simulink model "Full_drone_1_2"  (R2020b)
settings: Solver=VariableStepAuto  StartTime=0.0  StopTime=10  RelTol=1e-3
model workspace: external: MATLAB File C:\Users\maria\MATLAB\Projects\untitled\simscape_test\Full_drone_1_2_DataFile.m (data not in the file)
undefined symbols (not defined in the file or in its folder): b, CTgain, density, diameter, Jm, Ke, Kt, L, pitchKd, pitchKi, pitchKp, Rm, rollKd, rollKi, rollKp, smiData, X, xKd, xKi, xKp, xRef, Y, yawKd, yawKi, yawKp, yawRef, yKd, yKi, yKp, yRef, Z, zKd, zKi, zKp, zRef
libraries: sm_lib x75, fl_lib x23, nesl_utility x11
(part 1 of 2)
settings Model: Creator=jbmic  LastModifiedBy=maria

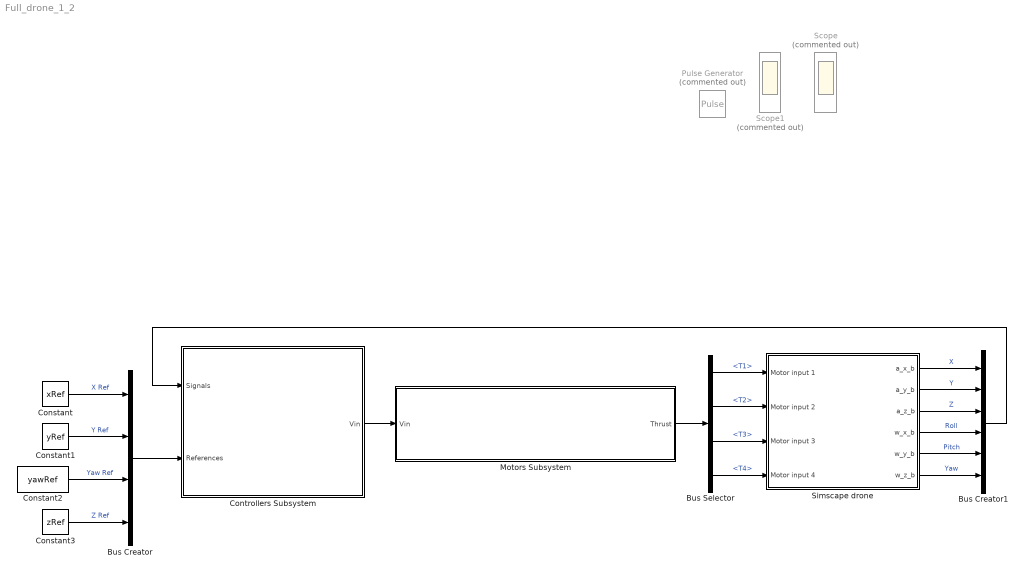
== system Full_drone_1_2 ==
  Bus Creator : BusCreator  Inputs=4
  Bus Creator1 : BusCreator  Inputs=6
  Bus Selector : BusSelector  OutputSignals=T1,T2,T3,T4
  Constant : Constant  Value=xRef
  Constant1 : Constant  Value=yRef
  Constant2 : Constant  Value=yawRef
  Constant3 : Constant  Value=zRef
  Controllers Subsystem : Subsystem
  Motors Subsystem : Subsystem
  Pulse Generator : DiscretePulseGenerator  Commented=on  PulseType=Time based  Amplitude=2  Period=1  PulseWidth=70
  Scope : Scope  Commented=on  NumInputPorts=3
  Scope1 : Scope  Commented=on  NumInputPorts=3
  Simscape drone : Subsystem
  wires:
  Simscape drone/4(w_x_b) -> Bus Creator1/4  "Roll"
  Simscape drone/5(w_y_b) -> Bus Creator1/5  "Pitch"
  Simscape drone/6(w_z_b) -> Bus Creator1/6  "Yaw"
  Simscape drone/3(a_z_b) -> Bus Creator1/3  "Z"
  Simscape drone/2(a_y_b) -> Bus Creator1/2  "Y"
  Simscape drone/1(a_x_b) -> Bus Creator1/1  "X"
  Bus Creator1/1 -> Controllers Subsystem/1(Signals)
  Constant/1 -> Bus Creator/1  "X Ref"
  Constant1/1 -> Bus Creator/2  "Y Ref"
  Constant2/1 -> Bus Creator/3  "Yaw Ref"
  Constant3/1 -> Bus Creator/4  "Z Ref"
  Bus Creator/1 -> Controllers Subsystem/2(References)
  Controllers Subsystem/1(Vin) -> Motors Subsystem/1(Vin)
  Motors Subsystem/1(Thrust) -> Bus Selector/1
  Bus Selector/3 -> Simscape drone/3(Motor input 3)  "<T3>"
  Bus Selector/4 -> Simscape drone/4(Motor input 4)  "<T4>"
  Bus Selector/2 -> Simscape drone/2(Motor input 2)  "<T2>"
  Bus Selector/1 -> Simscape drone/1(Motor input 1)  "<T1>"

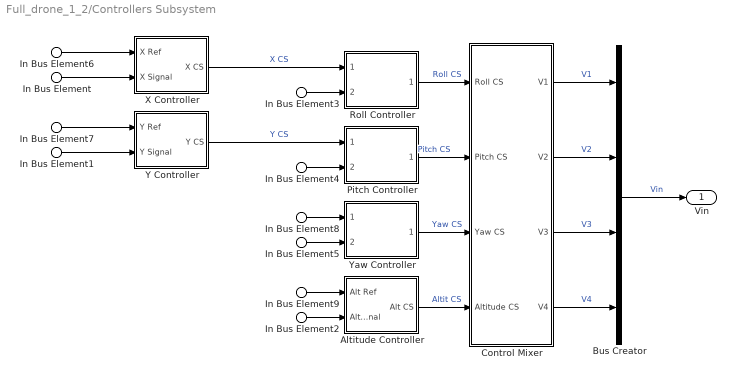
== system Full_drone_1_2/Controllers Subsystem ==
  In Bus Element : Inport  PortName=Signals  Element=X
  In Bus Element1 : Inport  PortName=Signals  Element=Y
  In Bus Element2 : Inport  PortName=Signals  Element=Z
  In Bus Element3 : Inport  PortName=Signals  Element=Roll
  In Bus Element4 : Inport  PortName=Signals  Element=Pitch
  In Bus Element5 : Inport  PortName=Signals  Element=Yaw
  In Bus Element6 : Inport  Port=2  PortName=References  Element=X Ref
  In Bus Element7 : Inport  Port=2  PortName=References  Element=Y Ref
  In Bus Element8 : Inport  Port=2  PortName=References  Element=Yaw Ref
  In Bus Element9 : Inport  Port=2  PortName=References  Element=Z Ref
  Altitude Controller : Subsystem
  Bus Creator : BusCreator  Inputs=4
  Control Mixer : Subsystem
  Pitch Controller : Subsystem
  Roll Controller : Subsystem
  X Controller : Subsystem
  Y Controller : Subsystem
  Yaw Controller : Subsystem
  Vin : Outport
  wires:
  In Bus Element9/1 -> Altitude Controller/1(Alt Ref)
  In Bus Element6/1 -> X Controller/1(X Ref)
  Control Mixer/3(V3) -> Bus Creator/3  "V3"
  In Bus Element8/1 -> Yaw Controller/1(Yaw Ref)
  Yaw Controller/1(Yaw CS) -> Control Mixer/3(Yaw CS)  "Yaw CS"
  In Bus Element7/1 -> Y Controller/1(Y Ref)
  Altitude Controller/1(Alt CS) -> Control Mixer/4(Altitude CS)  "Altit CS"
  X Controller/1(X CS) -> Roll Controller/1(Roll Ref)  "X CS"
  Y Controller/1(Y CS) -> Pitch Controller/1(Pitch Ref)  "Y CS"
  Pitch Controller/1(Pitch CS) -> Control Mixer/2(Pitch CS)  "Pitch CS"
  Control Mixer/2(V2) -> Bus Creator/2  "V2"
  Roll Controller/1(Roll CS) -> Control Mixer/1(Roll CS)  "Roll CS"
  Bus Creator/1 -> Vin/1  "Vin"
  Control Mixer/4(V4) -> Bus Creator/4  "V4"
  Control Mixer/1(V1) -> Bus Creator/1  "V1"
  In Bus Element/1 -> X Controller/2(X Signal)
  In Bus Element1/1 -> Y Controller/2(Y Signal)
  In Bus Element2/1 -> Altitude Controller/2(Alt Signal)
  In Bus Element3/1 -> Roll Controller/2(Roll Signal)
  In Bus Element4/1 -> Pitch Controller/2(Pitch Signal)
  In Bus Element5/1 -> Yaw Controller/2(Yaw Signal)

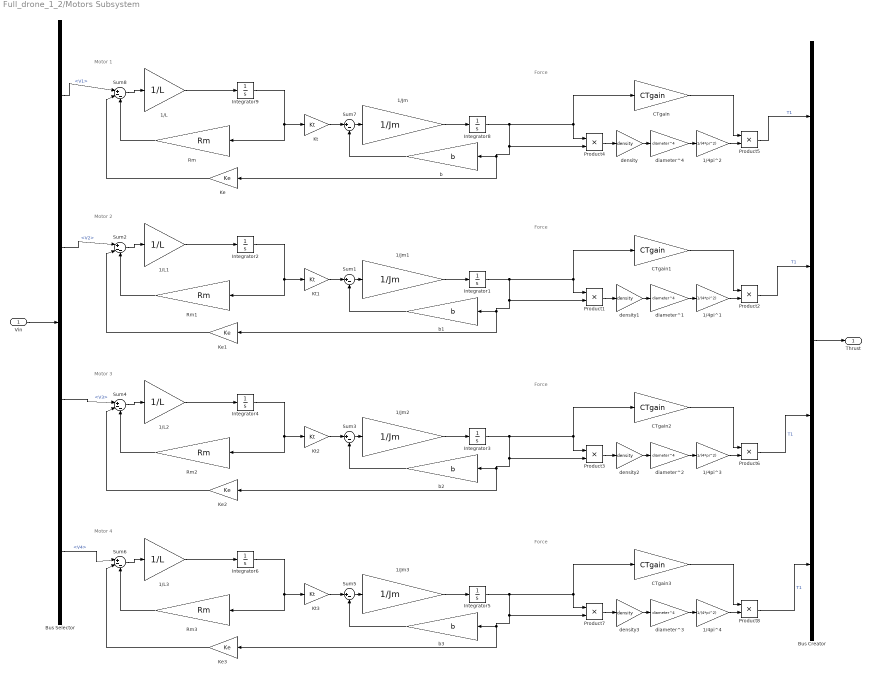
== system Full_drone_1_2/Motors Subsystem ==
  note: Motor 1
  note: Force
  note: Motor 2
  note: Force
  note: Motor 3
  note: Force
  note: Motor 4
  note: Force
  Vin : Inport
  1/4pi^{1..4} (4 alike) : Gain  Gain=1/(4*pi^2)
  1/Jm{,1..3} (4 alike) : Gain  Gain=1/Jm
  1/L{,1..3} (4 alike) : Gain  Gain=1/L
  Bus Creator : BusCreator  Inputs=4
  Bus Selector : BusSelector  OutputSignals=V1,V2,V3,V4
  CTgain{,1..3} (4 alike) : Gain  Gain=CTgain
  Integrator{1..6,8..9} (8 alike) : Integrator
  Ke{,1..3} (4 alike) : Gain  Gain=Ke
  Kt{,1..3} (4 alike) : Gain  Gain=Kt
  Product{1..8} (8 alike) : Product
  Rm{,1..3} (4 alike) : Gain  Gain=Rm
  Sum{1,3,5,7} (4 alike) : Sum  Inputs=|+-
  Sum{2,4,6,8} (4 alike) : Sum  Inputs=|+--
  b{,1..3} (4 alike) : Gain  Gain=b
  density{,1..3} (4 alike) : Gain  Gain=density
  diameter^{1..4} (4 alike) : Gain  Gain=diameter^4
  Thrust : Outport
  wires:
  Rm/1 -> Sum8/3
  1/L/1 -> Integrator9/1
  Sum7/1 -> 1/Jm/1
  density/1 -> diameter^4/1
  Integrator8/1 -> Ke/1, b/1, Product4/2, Product4/1, CTgain/1
  diameter^4/1 -> 1/4pi^2/1
  Ke/1 -> Sum8/2
  Product4/1 -> density/1
  Integrator9/1 -> Kt/1, Rm/1
  1/4pi^2/1 -> Product5/2
  Product5/1 -> Bus Creator/1  "T1"
  Bus Selector/1 -> Sum8/1  "<V1>"
  Sum8/1 -> 1/L/1
  Kt/1 -> Sum7/1
  1/Jm/1 -> Integrator8/1
  CTgain/1 -> Product5/1
  b/1 -> Sum7/2
  Vin/1 -> Bus Selector/1
  Bus Creator/1 -> Thrust/1
  Kt1/1 -> Sum1/1
  1/4pi^1/1 -> Product2/2
  diameter^1/1 -> 1/4pi^1/1
  1/L1/1 -> Integrator2/1
  Integrator1/1 -> Ke1/1, b1/1, Product1/2, Product1/1, CTgain1/1
  Product1/1 -> density1/1
  Ke1/1 -> Sum2/2
  Integrator2/1 -> Kt1/1, Rm1/1
  Sum2/1 -> 1/L1/1
  b1/1 -> Sum1/2
  CTgain1/1 -> Product2/1
  1/Jm1/1 -> Integrator1/1
  density1/1 -> diameter^1/1
  Rm1/1 -> Sum2/3
  Sum1/1 -> 1/Jm1/1
  Bus Selector/2 -> Sum2/1  "<V2>"
  Product2/1 -> Bus Creator/2  "T1"
  Kt2/1 -> Sum3/1
  1/4pi^3/1 -> Product6/2
  diameter^2/1 -> 1/4pi^3/1
  1/L2/1 -> Integrator4/1
  Integrator3/1 -> Ke2/1, b2/1, Product3/2, Product3/1, CTgain2/1
  Product3/1 -> density2/1
  Ke2/1 -> Sum4/2
  Integrator4/1 -> Kt2/1, Rm2/1
  Sum4/1 -> 1/L2/1
  b2/1 -> Sum3/2
  CTgain2/1 -> Product6/1
  1/Jm2/1 -> Integrator3/1
  density2/1 -> diameter^2/1
  Rm2/1 -> Sum4/3
  Sum3/1 -> 1/Jm2/1
  Bus Selector/3 -> Sum4/1  "<V3>"
  Product6/1 -> Bus Creator/3  "T1"
  Kt3/1 -> Sum5/1
  1/4pi^4/1 -> Product8/2
  diameter^3/1 -> 1/4pi^4/1
  1/L3/1 -> Integrator6/1
  Integrator5/1 -> Ke3/1, b3/1, Product7/2, Product7/1, CTgain3/1
  Product7/1 -> density3/1
  Ke3/1 -> Sum6/2
  Integrator6/1 -> Kt3/1, Rm3/1
  Sum6/1 -> 1/L3/1
  b3/1 -> Sum5/2
  CTgain3/1 -> Product8/1
  1/Jm3/1 -> Integrator5/1
  density3/1 -> diameter^3/1
  Rm3/1 -> Sum6/3
  Sum5/1 -> 1/Jm3/1
  Bus Selector/4 -> Sum6/1  "<V4>"
  Product8/1 -> Bus Creator/4  "T1"

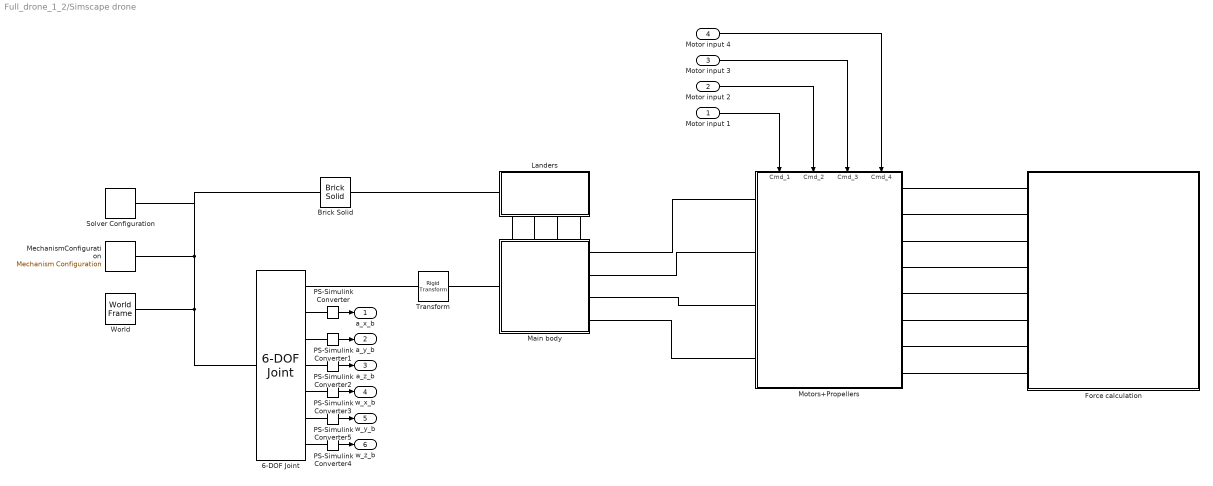
== system Full_drone_1_2/Simscape drone ==
  Motor input 1 : Inport
  Motor input 2 : Inport  Port=2
  Motor input 3 : Inport  Port=3
  Motor input 4 : Inport  Port=4
  6-DOF Joint : sm_lib/Joints/6-DOF Joint  JointMode=Normal  SenseConstraintForce=off  SenseConstraintForceX=off  SenseConstraintForceY=off  SenseConstraintForceZ=off  SenseConstraintTorque=off  SenseConstraintTorqueX=off  SenseConstraintTorqueY=off  SenseConstraintTorqueZ=off  SenseTotalForce=off  SenseTotalForceX=off  SenseTotalForceY=off  SenseTotalForceZ=off  SenseTotalTorque=off  SenseTotalTorqueX=off  SenseTotalTorqueY=off  SenseTotalTorqueZ=off  CompositeWrenchDir=FollowerOnBase  CompositeWrenchFrame=BaseFrame  PxEquilibriumPosition=0  PxEquilibriumPositionUnits=m  PxSpringStiffness=0  PxSpringStiffnessUnits=N/m  PxDampingCoefficient=0  PxDampingCoefficientUnits=N/(m/s)  PxTorqueActuationMode=NoTorque  PxMotionActuationMode=ComputedMotion  PxSensePosition=off  PxSenseVelocity=off  PxSenseAcceleration=on  PxSenseTorqueForce=off  PxSenseLowerLimitTorqueForce=off  PxSenseUpperLimitTorqueForce=off  PxLowerLimitSpecify=off  PxLowerLimitBound=-1  PxLowerLimitBoundUnits=m  PxLowerLimitStiffness=1e6  PxLowerLimitStiffnessUnits=N/m  PxLowerLimitDamping=1e3  PxLowerLimitDampingUnits=N/(m/s)  PxLowerLimitTransitionRegionWidth=1e-4  PxLowerLimitTransitionRegionWidthUnits=m  PxUpperLimitSpecify=off  PxUpperLimitBound=1  PxUpperLimitBoundUnits=m  PxUpperLimitStiffness=1e6  PxUpperLimitStiffnessUnits=N/m  PxUpperLimitDamping=1e3  PxUpperLimitDampingUnits=N/(m/s)  PxUpperLimitTransitionRegionWidth=1e-4  PxUpperLimitTransitionRegionWidthUnits=m  PxPositionTargetSpecify=off  PxPositionTargetPriority=High  PxPositionTargetValue=0  PxPositionTargetValueUnits=m  PxVelocityTargetSpecify=off  PxVelocityTargetPriority=High  PxVelocityTargetValue=0  PxVelocityTargetValueUnits=m/s  PyEquilibriumPosition=0  PyEquilibriumPositionUnits=m  PySpringStiffness=0  PySpringStiffnessUnits=N/m  PyDampingCoefficient=0  PyDampingCoefficientUnits=N/(m/s)  PyTorqueActuationMode=NoTorque  PyMotionActuationMode=ComputedMotion  PySensePosition=off  PySenseVelocity=off  PySenseAcceleration=on  PySenseTorqueForce=off  PySenseLowerLimitTorqueForce=off  PySenseUpperLimitTorqueForce=off  PyLowerLimitSpecify=off  PyLowerLimitBound=0  PyLowerLimitBoundUnits=m  PyLowerLimitStiffness=1e6  PyLowerLimitStiffnessUnits=N/m  PyLowerLimitDamping=1  PyLowerLimitDampingUnits=N/(m/s)  PyLowerLimitTransitionRegionWidth=1e4  PyLowerLimitTransitionRegionWidthUnits=m  PyUpperLimitSpecify=off  PyUpperLimitBound=1  PyUpperLimitBoundUnits=m  PyUpperLimitStiffness=1e6  PyUpperLimitStiffnessUnits=N/m  PyUpperLimitDamping=1e3  PyUpperLimitDampingUnits=N/(m/s)  PyUpperLimitTransitionRegionWidth=1e-4  PyUpperLimitTransitionRegionWidthUnits=m  PyPositionTargetSpecify=off  PyPositionTargetPriority=High  PyPositionTargetValue=0  PyPositionTargetValueUnits=m  PyVelocityTargetSpecify=off  PyVelocityTargetPriority=High  PyVelocityTargetValue=0  PyVelocityTargetValueUnits=m/s  PzEquilibriumPosition=0  PzEquilibriumPositionUnits=m  PzSpringStiffness=0  PzSpringStiffnessUnits=N/m  PzDampingCoefficient=0  PzDampingCoefficientUnits=N/(m/s)  PzTorqueActuationMode=NoTorque  PzMotionActuationMode=ComputedMotion  PzSensePosition=off  PzSenseVelocity=off  PzSenseAcceleration=on  PzSenseTorqueForce=off  PzSenseLowerLimitTorqueForce=off  PzSenseUpperLimitTorqueForce=off  PzLowerLimitSpecify=off  PzLowerLimitBound=-1  PzLowerLimitBoundUnits=m  PzLowerLimitStiffness=1e6  PzLowerLimitStiffnessUnits=N/m  PzLowerLimitDamping=1e3  PzLowerLimitDampingUnits=N/(m/s)  PzLowerLimitTransitionRegionWidth=1e-4  PzLowerLimitTransitionRegionWidthUnits=m  PzUpperLimitSpecify=off  PzUpperLimitBound=1  PzUpperLimitBoundUnits=m  PzUpperLimitStiffness=1e6  PzUpperLimitStiffnessUnits=N/m  PzUpperLimitDamping=1e3  PzUpperLimitDampingUnits=N/(m/s)  PzUpperLimitTransitionRegionWidth=1e-4  PzUpperLimitTransitionRegionWidthUnits=m  PzPositionTargetSpecify=off  PzPositionTargetPriority=High  PzPositionTargetValue=0  PzPositionTargetValueUnits=m  PzVelocityTargetSpecify=off  PzVelocityTargetPriority=High  PzVelocityTargetValue=0  PzVelocityTargetValueUnits=m/s  SphDefPosRotationMethod=None  SphDefPosRotationAngleUnits=deg  SphDefPosRotationStandardAxis=+Z  SphDefPosRotationAngle=0.0  SphDefPosRotationArbitraryAxis=[0 0 1]  SphDefPosFollAlignAxisA=+X  SphDefPosBaseAlignAxisA=+Y  SphDefPosFollAlignAxisB=+Y  SphDefPosBaseAlignAxisB=+Z  SphDefPosRotationSequenceAxes=FollowerAxes  SphDefPosRotationSequence=XYX  SphDefPosRotationSequenceAngles=[0 0 0]  SphDefPosRotationSequenceAnglesUnits=deg  SphDefPosRotationMatrix=[1 0 0; 0 1 0; 0 0 1]  SphEqPosRotationMethod=None  SphEqPosRotationAngleUnits=deg  SphEqPosRotationStandardAxis=+Z  SphEqPosRotationAngle=0.0  SphEqPosRotationArbitraryAxis=[0 0 1]  SphEqPosFollAlignAxisA=+X  SphEqPosBaseAlignAxisA=+Y  SphEqPosFollAlignAxisB=+Y  SphEqPosBaseAlignAxisB=+Z  SphEqPosRotationSequenceAxes=FollowerAxes  SphEqPosRotationSequence=XYX  SphEqPosRotationSequenceAngles=[0 0 0]  SphEqPosRotationSequenceAnglesUnits=deg  SphEqPosRotationMatrix=[1 0 0; 0 1 0; 0 0 1]  SphSpringStiffness=0  SphSpringStiffnessUnits=N*m/deg  SphDampingCoefficient=1e-2  SphDampingCoefficientUnits=N*m/(deg/s)  SphActuateTorqueX=off  SphActuateTorqueY=off  SphActuateTorqueZ=off  SphActuateTorque=off  SphTorqueActuationMode=NoTorque  SphMotionActuationMode=ComputedMotion  SphActuationFrame=BaseFrame  SphSensePosition=off  SphSenseVelocityX=on  SphSenseVelocityY=on  SphSenseVelocityZ=on  SphSenseVelocity=off  SphSenseAccelerationX=off  SphSenseAccelerationY=off  SphSenseAccelerationZ=off  SphSenseAcceleration=off  SphSenseTorqueX=off  SphSenseTorqueY=off  SphSenseTorqueZ=off  SphSenseTorqueForce=off  SphSenseLowerLimitTorqueMag=off  SphSenseUpperLimitTorqueMag=off  SphSensingFrame=BaseFrame  SphLowerLimitSpecify=off  SphLowerLimitBound=15  SphLowerLimitBoundUnits=deg  SphLowerLimitStiffness=1e4  SphLowerLimitStiffnessUnits=N*m/deg  SphLowerLimitDamping=10  SphLowerLimitDampingUnits=N*m/(deg/s)  SphLowerLimitTransitionRegionWidth=0.1  SphLowerLimitTransitionRegionWidthUnits=deg  SphUpperLimitSpecify=off  SphUpperLimitBound=45  SphUpperLimitBoundUnits=deg  SphUpperLimitStiffness=1e4  SphUpperLimitStiffnessUnits=N*m/deg  SphUpperLimitDamping=10  SphUpperLimitDampingUnits=N*m/(deg/s)  SphUpperLimitTransitionRegionWidth=0.1  SphUpperLimitTransitionRegionWidthUnits=deg  SphPositionTargetRotationMethod=None  SphPositionTargetRotationAngleUnits=deg  SphPositionTargetRotationStandardAxis=+Z  SphPositionTargetRotationAngle=0.0  SphPositionTargetRotationArbitraryAxis=[0 0 1]  SphPositionTargetFollAlignAxisA=+X  SphPositionTargetBaseAlignAxisA=+Y  SphPositionTargetFollAlignAxisB=+Y  SphPositionTargetBaseAlignAxisB=+Z  SphPositionTargetRotationSequenceAxes=FollowerAxes  SphPositionTargetRotationSequence=XYX  SphPositionTargetRotationSequenceAngles=[0 0 0]  SphPositionTargetRotationSequenceAnglesUnits=deg  SphPositionTargetRotationMatrix=[1 0 0; 0 1 0; 0 0 1]  SphPositionTargetSpecify=off  SphPositionTargetPriority=High  SphVelocityTargetValue=[0 0 0]  SphVelocityTargetValueUnits=deg/s  SphVelocityTargetSpecify=off  SphVelocityTargetPriority=High  SphVelocityTargetInFollowerFrame=on
  Brick Solid : sm_lib/Body Elements/Brick Solid  GraphicAmbientColor=[0.15 0.15 0.15 1.0]  BasedOnType=Density  BrickDimensions=[1 1 0.002]  BrickDimensionUnits=m  CenterOfMass=[0 0 0]  CenterOfMassUnits=m  GraphicDiffuseColor=[0.5 0.5 0.5]  Density=1000  DensityUnits=kg/m^3  DoExposeReferenceFrame=on  GraphicEmissiveColor=[0.0 0.0 0.0 1.0]  ExportEntireGeometry=on  SerializedFrames=<Frames/>  MarkerShape=Sphere  MarkerSize=10  GraphicType=FromGeometry  InertiaType=CalculateFromGeometry  Mass=1  MassUnits=kg  MomentsOfInertia=[1 1 1]  MomentsOfInertiaUnits=kg*m^2  GraphicOpacity=1.0  ProductsOfInertia=[0 0 0]  ProductsOfInertiaUnits=kg*m^2  GraphicShininess=75  GraphicSpecularColor=[0.5 0.5 0.5 1.0]  GraphicVisPropType=SimpleVisualProperties
  Force calculation : Subsystem
  Landers : Subsystem
      settings: PortSchema="{\"entries\":[{\"content\":{\"sides\":[{\"content\":{\"connectorIds\":[]},\"type\":\"ConnectorPlacement.EquallySpacedRectSide\",\"uuid\":\"29ed25fe-b3f0-40d8-8e38-dad31f47c1c2\"},{\"content\":{\"connectorIds\":[\"RConn1\"],\"side\":\"RIGHT\"},\"type\":\"ConnectorPlacement.EquallySpacedRectSide\",\"uuid\":\"a44326be-c514-4699-a20f-f031abb9163a\"},{\"content\":{\"connectorIds\":[\"LConn1\",\"LConn2\",\"LConn3\",\"LConn4\"],\"side\":\"TOP\"},\"type\":\"ConnectorPlacement.EquallySpacedRectSide\",\"uuid\":\"e989b3f4-324c-4714-b27e-b8d073d4c35f\"},{\"content\":{\"connectorIds\":[],\"side\":\"HIDDEN\"},\"type\":\"ConnectorPlacement.EquallySpacedRectSide\",\"uuid\":\"003ab62d-37b6-4b48-957b-1f2b95d598b0\"}]},\"type\":\"ConnectorPlacement.EquallySpacedConnector\",\"uuid\":\"ee59c263-ccee-4526-9944-481878d464b1\"}],\"packageUris\":[\"http://schema.mathworks.com/mf0/Connector/R2020b\"],\"version\":\"1.0\"}"
  Main body : Subsystem
      settings: PortSchema="{\"entries\":[{\"content\":{\"sides\":[{\"content\":{\"connectorIds\":[\"LConn1\"]},\"type\":\"ConnectorPlacement.EquallySpacedRectSide\",\"uuid\":\"1d560889-63f6-48ae-9785-9ad03b6228cb\"},{\"content\":{\"connectorIds\":[\"RConn1\",\"RConn2\",\"RConn3\",\"RConn4\"],\"side\":\"RIGHT\"},\"type\":\"ConnectorPlacement.EquallySpacedRectSide\",\"uuid\":\"3b5eeccf-6620-4e96-a65e-dc2a1dbf3c1a\"},{\"content\":{\"connectorIds\":[\"LConn2\",\"LConn3\",\"LConn4\",\"LConn5\"],\"side\":\"TOP\"},\"type\":\"ConnectorPlacement.EquallySpacedRectSide\",\"uuid\":\"c37c81f4-9ca5-430c-b06e-204f4de6e523\"},{\"content\":{\"connectorIds\":[],\"side\":\"BOTTOM\"},\"type\":\"ConnectorPlacement.EquallySpacedRectSide\",\"uuid\":\"a07765c1-544d-4fcc-9081-a11d0d1876aa\"},{\"content\":{\"connectorIds\":[],\"side\":\"HIDDEN\"},\"type\":\"ConnectorPlacement.EquallySpacedRectSide\",\"uuid\":\"1cae8fd9-d51c-4e2a-9399-ab36badad5a4\"}]},\"type\":\"ConnectorPlacement.EquallySpacedConnector\",\"uuid\":\"00156c8e-efff-419c-9276-6474ba4529e4\"}],\"packageUris\":[\"http://schema.mathworks.com/mf0/Connector/R2020b\"],\"version\":\"1.0\"}"
  MechanismConfiguration : sm_lib/Utilities/Mechanism Configuration  UniformGravity=Constant  GravityVector=[0 0 -9.81]  GravityVectorUnits=m/s^2  GravityUnits=m/s^2  LinearizationDelta=0.001  JointModeTransitionNonlinearIterations=2
  Motors+Propellers : Subsystem
      settings: PortSchema="{\"entries\":[{\"content\":{\"sides\":[{\"content\":{\"connectorIds\":[\"LConn1\",\"LConn2\",\"LConn3\",\"LConn4\"]},\"type\":\"ConnectorPlacement.EquallySpacedRectSide\",\"uuid\":\"a87e523b-4188-4a06-84bc-a56bd0d2fcc6\"},{\"content\":{\"connectorIds\":[\"RConn1\",\"RConn2\",\"RConn3\",\"RConn4\",\"RConn5\",\"RConn6\",\"RConn7\",\"RConn8\"],\"side\":\"RIGHT\"},\"type\":\"ConnectorPlacement.EquallySpacedRectSide\",\"uuid\":\"8bc1e91e-dcc0-4c0e-875b-f0693b226b59\"},{\"content\":{\"connectorIds\":[\"In1\",\"In2\",\"In3\",\"In4\"],\"side\":\"TOP\"},\"type\":\"ConnectorPlacement.EquallySpacedRectSide\",\"uuid\":\"30d4fa00-3250-4c05-889a-a7c5558f86c5\"},{\"content\":{\"connectorIds\":[],\"side\":\"BOTTOM\"},\"type\":\"ConnectorPlacement.EquallySpacedRectSide\",\"uuid\":\"383305d0-285c-429a-9b45-ff468c120a62\"},{\"content\":{\"connectorIds\":[],\"side\":\"HIDDEN\"},\"type\":\"ConnectorPlacement.EquallySpacedRectSide\",\"uuid\":\"8700f3ae-88a9-49c8-857d-0b2e7efcfe18\"}]},\"type\":\"ConnectorPlacement.EquallySpacedConnector\",\"uuid\":\"10251bd4-0e37-45aa-b66f-3df2db35b3c6\"}],\"packageUris\":[\"http://schema.mathworks.com/mf0/Connector/R2020b\"],\"version\":\"1.0\"}"
  PS-Simulink Converter{,1..5} (6 alike) : nesl_utility/PS-Simulink Converter  PhysicalDomain=network_engine_domain  SubClassName=ps_output  LeftPortType=input  RightPortType=output  PseudoPeriodic=off  Frequencies=[]  Unit=inherit  AffineConversion=off
  Solver Configuration : nesl_utility/Solver Configuration  PhysicalDomain=network_engine_domain  SubClassName=solver  LeftPortType=input  RightPortType=generic  Tones=[]  Harmonics=[]  SimulateNoise=off  Profile=off  UseLocalSampling=off  EnableSwitchedLinearOptims=on  FrequencyDomain=off  UseCCode=off  RelTol=0.001  AbsTol=1e-06  MinStep=1e-09  ToWorkspace=off  RevertToSquareIcSolve=off  NumHomotopyIterations=100  PhasorMode=off  PhasorModeNumHarmonics=1  DoDC=off  ResidualTolerance=1e-09  UseLocalSolver=off  LocalSolverChoice=NE_BACKWARD_EULER_ADVANCER  LocalSolverSampleTime=0.001  DoFixedCost=off  MaxNonlinIter=3  MaxModeIter=2  ComputeImpulses=off  ImpulseIterations=2  LinearAlgebra=auto  EquationFormulation=NE_TIME_EF  DelaysMemoryBudget=1024  AutomaticFiltering=on  FilteringTimeConstant=0.001  PartitionStorageMethod=AS_NEEDED  PartitionMemoryBudget=1024  PartitionMethod=ROBUST
  Transform : sm_lib/Frames and Transforms/Rigid Transform  TranslationMethod=Cartesian  TranslationStandardOffset=100  TranslationLengthUnit=mm  TranslationStandardAxis=+Z  TranslationCartesianOffset=smiData.RigidTransform(27).translation  TranslationROffset=0  TranslationROffsetUnits=m  TranslationZOffset=0  TranslationZOffsetUnits=m  TranslationThetaOffset=0  TranslationThetaOffsetUnits=deg  RotationMethod=StandardAxis  RotationAngleUnits=deg  RotationStandardAxis=+X  RotationAngle=90  RotationArbitraryAxis=smiData.RigidTransform(27).axis  FollAlignAxisA=+X  BaseAlignAxisA=+Y  FollAlignAxisB=+Y  BaseAlignAxisB=+Z  RotationSequenceAxes=FollowerAxes  RotationSequence=XYX  RotationSequenceAngles=[0 0 0]  RotationSequenceAnglesUnits=deg  RotationMatrix=[1 0 0; 0 1 0; 0 0 1]
  World : sm_lib/Frames and Transforms/World Frame
  a_x_b : Outport
  a_y_b : Outport  Port=2
  a_z_b : Outport  Port=3
  w_x_b : Outport  Port=4
  w_y_b : Outport  Port=5
  w_z_b : Outport  Port=6
  wires:
  Motor input 1/1 -> Motors+Propellers/1(Cmd_1)
  Motor input 2/1 -> Motors+Propellers/2(Cmd_2)
  Motor input 3/1 -> Motors+Propellers/3(Cmd_3)
  Motor input 4/1 -> Motors+Propellers/4(Cmd_4)
  PS-Simulink Converter/1 -> a_x_b/1
  PS-Simulink Converter1/1 -> a_y_b/1
  PS-Simulink Converter2/1 -> a_z_b/1
  PS-Simulink Converter3/1 -> w_x_b/1
  PS-Simulink Converter5/1 -> w_y_b/1
  PS-Simulink Converter4/1 -> w_z_b/1
  connections:
  Force calculation/LConn8 -- Motors+Propellers/RConn8
  MechanismConfiguration/RConn1 -- Brick Solid/RConn1 -- Solver Configuration/RConn1 -- World/RConn1 -- 6-DOF Joint/LConn1
  Motors+Propellers/LConn4 -- Main body/RConn4
  Force calculation/LConn6 -- Motors+Propellers/RConn6
  6-DOF Joint/RConn1 -- Transform/LConn1
  Motors+Propellers/LConn2 -- Main body/RConn2
  Motors+Propellers/LConn3 -- Main body/RConn3
  Force calculation/LConn3 -- Motors+Propellers/RConn3
  Motors+Propellers/LConn1 -- Main body/RConn1
  Force calculation/LConn7 -- Motors+Propellers/RConn7
  Motors+Propellers/RConn1 -- Force calculation/LConn1
  Transform/RConn1 -- Main body/LConn1
  Force calculation/LConn2 -- Motors+Propellers/RConn2
  Force calculation/LConn5 -- Motors+Propellers/RConn5
  Motors+Propellers/RConn4 -- Force calculation/LConn4
  Landers/LConn4 -- Main body/LConn2
  Landers/LConn3 -- Main body/LConn3
  Landers/LConn2 -- Main body/LConn4
  Landers/LConn1 -- Main body/LConn5
  Brick Solid/LConn1 -- Landers/RConn1
  PS-Simulink Converter/LConn1 -- 6-DOF Joint/RConn2
  PS-Simulink Converter1/LConn1 -- 6-DOF Joint/RConn3
  PS-Simulink Converter5/LConn1 -- 6-DOF Joint/RConn6
  PS-Simulink Converter3/LConn1 -- 6-DOF Joint/RConn5
  6-DOF Joint/RConn4 -- PS-Simulink Converter2/LConn1
  6-DOF Joint/RConn7 -- PS-Simulink Converter4/LConn1

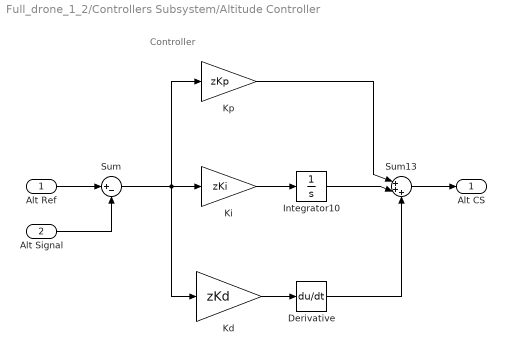
== system Full_drone_1_2/Controllers Subsystem/Altitude Controller ==
  note: Controller
  Alt Ref : Inport
  Alt Signal : Inport  Port=2
  Derivative : Derivative
  Integrator10 : Integrator
  "Kd " : Gain  Gain=zKd
  Ki : Gain  Gain=zKi
  Kp : Gain  Gain=zKp
  Sum : Sum  Inputs=|+-
  Sum13 : Sum  Inputs=|+++
  Alt CS : Outport
  wires:
  Derivative/1 -> Sum13/3
  Ki/1 -> Integrator10/1
  Integrator10/1 -> Sum13/2
  Kp/1 -> Sum13/1
  "Kd "/1 -> Derivative/1
  Sum13/1 -> Alt CS/1
  Alt Ref/1 -> Sum/1
  Alt Signal/1 -> Sum/2
  Sum/1 -> Kp/1, "Kd "/1, Ki/1

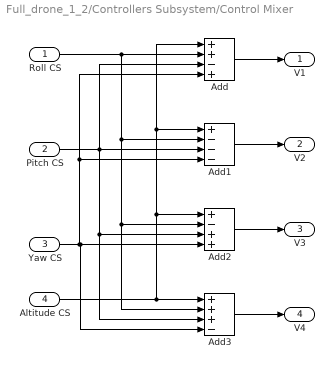
== system Full_drone_1_2/Controllers Subsystem/Control Mixer ==
  Roll CS : Inport
  Pitch CS : Inport  Port=2
  Yaw CS : Inport  Port=3
  Altitude CS : Inport  Port=4
  Add : Sum  Inputs=++-+
  Add1 : Sum  Inputs=+---
  Add2 : Sum  Inputs=+-++
  Add3 : Sum  Inputs=+++-
  V1 : Outport
  V2 : Outport  Port=2
  V3 : Outport  Port=3
  V4 : Outport  Port=4
  wires:
  Add/1 -> V1/1
  Add1/1 -> V2/1
  Add3/1 -> V4/1
  Add2/1 -> V3/1
  Altitude CS/1 -> Add2/1, Add1/1, Add/1, Add3/1
  Roll CS/1 -> Add1/2, Add2/2, Add3/2, Add/2
  Pitch CS/1 -> Add3/3, Add2/3, Add/3, Add1/3
  Yaw CS/1 -> Add/4, Add1/4, Add3/4, Add2/4

== system Full_drone_1_2/Controllers Subsystem/Pitch Controller ==
  note: Controller
  Pitch Ref : Inport
  Pitch Signal : Inport  Port=2
  Derivative : Derivative
  Integrator10 : Integrator
  Kd : Gain  Gain=pitchKd
  Ki : Gain  Gain=pitchKi
  Kp : Gain  Gain=pitchKp
  Sum : Sum  Inputs=|+-
  Sum13 : Sum  Inputs=|+++
  Pitch CS : Outport
  wires:
  Derivative/1 -> Sum13/3
  Ki/1 -> Integrator10/1
  Integrator10/1 -> Sum13/2
  Kp/1 -> Sum13/1
  Kd/1 -> Derivative/1
  Sum13/1 -> Pitch CS/1
  Pitch Ref/1 -> Sum/1
  Pitch Signal/1 -> Sum/2
  Sum/1 -> Kd/1, Ki/1, Kp/1

== system Full_drone_1_2/Controllers Subsystem/Roll Controller ==
  note: Controller
  Roll Ref : Inport
  Roll Signal : Inport  Port=2
  Derivative : Derivative
  Integrator10 : Integrator
  Kd : Gain  Gain=rollKd
  Ki : Gain  Gain=rollKi
  Kp : Gain  Gain=rollKp
  Sum : Sum  Inputs=|+-
  Sum13 : Sum  Inputs=|+++
  Roll CS : Outport
  wires:
  Derivative/1 -> Sum13/3
  Ki/1 -> Integrator10/1
  Integrator10/1 -> Sum13/2
  Kp/1 -> Sum13/1
  Kd/1 -> Derivative/1
  Sum13/1 -> Roll CS/1
  Roll Ref/1 -> Sum/1
  Roll Signal/1 -> Sum/2
  Sum/1 -> Ki/1, Kp/1, Kd/1

== system Full_drone_1_2/Controllers Subsystem/X Controller ==
  note: Controller
  X Ref : Inport
  X Signal : Inport  Port=2
  Derivative : Derivative
  Integrator10 : Integrator
  Kd : Gain  Gain=xKd
  Ki : Gain  Gain=xKi
  Kp : Gain  Gain=xKp
  Sum : Sum  Inputs=|+-
  Sum13 : Sum  Inputs=|+++
  X CS : Outport
  wires:
  Derivative/1 -> Sum13/3
  Ki/1 -> Integrator10/1
  Integrator10/1 -> Sum13/2
  Kp/1 -> Sum13/1
  Kd/1 -> Derivative/1
  Sum13/1 -> X CS/1
  X Ref/1 -> Sum/1
  X Signal/1 -> Sum/2
  Sum/1 -> Kd/1, Kp/1, Ki/1

== system Full_drone_1_2/Controllers Subsystem/Y Controller ==
  note: Controller
  Y Ref : Inport
  Y Signal : Inport  Port=2
  Derivative : Derivative
  Integrator10 : Integrator
  Kd : Gain  Gain=yKd
  Ki : Gain  Gain=yKi
  Kp : Gain  Gain=yKp
  Sum : Sum  Inputs=|+-
  Sum13 : Sum  Inputs=|+++
  Y CS : Outport
  wires:
  Derivative/1 -> Sum13/3
  Ki/1 -> Integrator10/1
  Integrator10/1 -> Sum13/2
  Kp/1 -> Sum13/1
  Kd/1 -> Derivative/1
  Sum13/1 -> Y CS/1
  Y Ref/1 -> Sum/1
  Y Signal/1 -> Sum/2
  Sum/1 -> Kd/1, Kp/1, Ki/1

== system Full_drone_1_2/Controllers Subsystem/Yaw Controller ==
  note: Controller
  Yaw Ref : Inport
  Yaw Signal : Inport  Port=2
  Derivative : Derivative
  Integrator10 : Integrator
  Kd : Gain  Gain=yawKd
  Ki : Gain  Gain=yawKi
  Kp : Gain  Gain=yawKp
  Sum : Sum  Inputs=|+-
  Sum13 : Sum  Inputs=|+++
  Yaw CS : Outport
  wires:
  Derivative/1 -> Sum13/3
  Ki/1 -> Integrator10/1
  Integrator10/1 -> Sum13/2
  Kp/1 -> Sum13/1
  Kd/1 -> Derivative/1
  Sum13/1 -> Yaw CS/1
  Yaw Ref/1 -> Sum/1
  Yaw Signal/1 -> Sum/2
  Sum/1 -> Ki/1, Kp/1, Kd/1

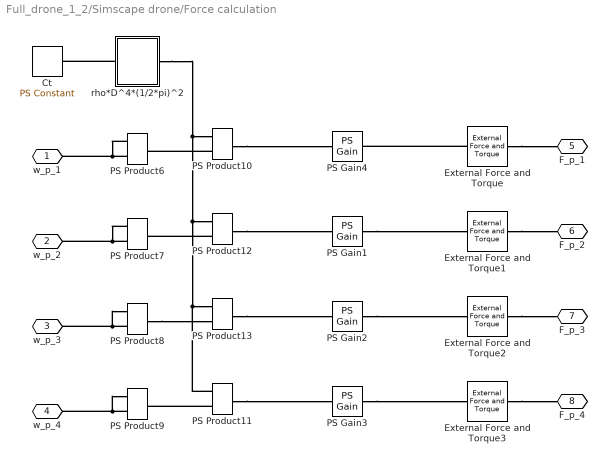
== system Full_drone_1_2/Simscape drone/Force calculation ==
  Ct : fl_lib/Physical Signals/Sources/PS Constant  constant=1
  External Force and Torque{,1..3} (4 alike) : sm_lib/Forces and Torques/External Force and Torque  ForceResolutionFrame=AttachedFrame  EnableForceX=off  EnableForceY=off  EnableForceZ=on  EnableForce=off  TorqueResolutionFrame=AttachedFrame  EnableTorqueX=off  EnableTorqueY=off  EnableTorqueZ=off  EnableTorque=off
  PS Gain1 : fl_lib/Physical Signals/Functions/PS Gain  gain=-1
  PS Gain2 : fl_lib/Physical Signals/Functions/PS Gain  gain=1
  PS Gain3 : fl_lib/Physical Signals/Functions/PS Gain  gain=-1
  PS Gain4 : fl_lib/Physical Signals/Functions/PS Gain  gain=-1
  PS Product{6..13} (8 alike) : fl_lib/Physical Signals/Functions/PS Product
  rho*D^4*(1/2*pi)^2 : Subsystem
  w_p_1 : PMIOPort  Side=Left
  w_p_2 : PMIOPort  Port=2  Side=Left
  w_p_3 : PMIOPort  Port=3  Side=Left
  w_p_4 : PMIOPort  Port=4  Side=Left
  F_p_1 : PMIOPort  Port=5  Side=Left
  F_p_2 : PMIOPort  Port=6  Side=Left
  F_p_3 : PMIOPort  Port=7  Side=Left
  F_p_4 : PMIOPort  Port=8  Side=Left
  connections:
  External Force and Torque2/RConn1 -- F_p_3/RConn1
  External Force and Torque/RConn1 -- F_p_1/RConn1
  External Force and Torque1/RConn1 -- F_p_2/RConn1
  External Force and Torque3/RConn1 -- F_p_4/RConn1
  PS Product6/LConn2 -- PS Product6/LConn1 -- w_p_1/RConn1
  PS Product7/LConn2 -- PS Product7/LConn1 -- w_p_2/RConn1
  PS Product8/LConn2 -- PS Product8/LConn1 -- w_p_3/RConn1
  PS Product9/LConn2 -- PS Product9/LConn1 -- w_p_4/RConn1
  PS Product10/LConn2 -- PS Product6/RConn1
  PS Product11/LConn2 -- PS Product9/RConn1
  PS Product12/LConn2 -- PS Product7/RConn1
  PS Product8/RConn1 -- PS Product13/LConn2
  rho*D^4*(1/2*pi)^2/LConn1 -- Ct/RConn1
  rho*D^4*(1/2*pi)^2/RConn1 -- PS Product11/LConn1 -- PS Product13/LConn1 -- PS Product12/LConn1 -- PS Product10/LConn1
  External Force and Torque/LConn1 -- PS Gain4/RConn1
  PS Gain1/RConn1 -- External Force and Torque1/LConn1
  PS Gain2/RConn1 -- External Force and Torque2/LConn1
  PS Gain3/RConn1 -- External Force and Torque3/LConn1
  PS Product10/RConn1 -- PS Gain4/LConn1
  PS Product12/RConn1 -- PS Gain1/LConn1
  PS Product13/RConn1 -- PS Gain2/LConn1
  PS Product11/RConn1 -- PS Gain3/LConn1

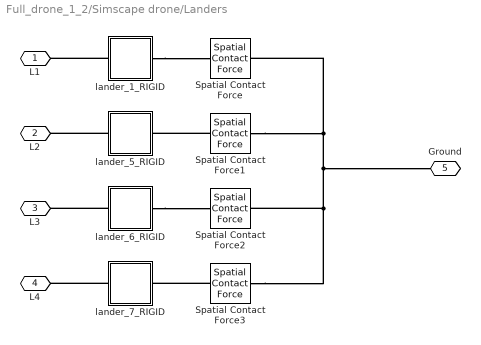
== system Full_drone_1_2/Simscape drone/Landers ==
  Spatial Contact Force{,1..3} (4 alike) : sm_lib/Forces and Torques/Spatial Contact Force  CoefficientOfDynamicFriction=0.3  CoefficientOfStaticFriction=0.5  NormalDamping=3e2  NormalDampingUnits=N/(m/s)  NormalStiffness=1e6  NormalStiffnessUnits=N/m  FrictionalCriticalVelocity=1e-3  FrictionalCriticalVelocityUnits=m/s  ZeroCrossDetectContactStartAndEnd=off  SenseFrictionalForceMagnitude=off  SenseNormalForceMagnitude=off  SenseSeparationDistance=off  NormalTransitionRegionWidth=1e-4  NormalTransitionRegionWidthUnits=m  FrictionType=SmoothStickSlip
  lander_1_RIGID : Subsystem
  lander_5_RIGID : Subsystem
  lander_6_RIGID : Subsystem
  lander_7_RIGID : Subsystem
  L1 : PMIOPort  Side=Left
  L2 : PMIOPort  Port=2  Side=Left
  L3 : PMIOPort  Port=3  Side=Left
  L4 : PMIOPort  Port=4  Side=Left
  Ground : PMIOPort  Port=5  Side=Right
  connections:
  lander_7_RIGID/LConn1 -- L4/RConn1
  lander_5_RIGID/LConn1 -- L2/RConn1
  lander_1_RIGID/LConn1 -- L1/RConn1
  lander_6_RIGID/LConn1 -- L3/RConn1
  lander_1_RIGID/RConn1 -- Spatial Contact Force/LConn1
  Spatial Contact Force1/LConn1 -- lander_5_RIGID/RConn1
  Spatial Contact Force3/RConn1 -- Spatial Contact Force2/RConn1 -- Spatial Contact Force1/RConn1 -- Spatial Contact Force/RConn1 -- Ground/RConn1
  lander_6_RIGID/RConn1 -- Spatial Contact Force2/LConn1
  Spatial Contact Force3/LConn1 -- lander_7_RIGID/RConn1

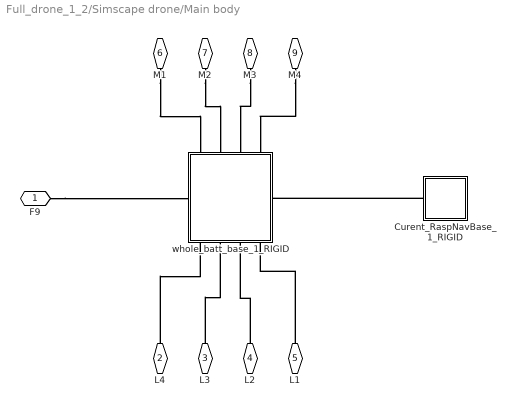
== system Full_drone_1_2/Simscape drone/Main body ==
  Curent_RaspNavBase_1_RIGID : Subsystem
  whole_batt_base_1_RIGID : Subsystem
      settings: PortSchema="{\"entries\":[{\"content\":{\"sides\":[{\"content\":{\"connectorIds\":[\"LConn1\"]},\"type\":\"ConnectorPlacement.EquallySpacedRectSide\",\"uuid\":\"3b6cc577-d81e-4bf8-866b-02a223ee5ba0\"},{\"content\":{\"connectorIds\":[\"RConn1\"],\"side\":\"RIGHT\"},\"type\":\"ConnectorPlacement.EquallySpacedRectSide\",\"uuid\":\"154d185d-d80c-4e9f-a785-b85ba4894acd\"},{\"content\":{\"connectorIds\":[\"LConn2\",\"LConn3\",\"LConn4\",\"LConn5\"],\"side\":\"TOP\"},\"type\":\"ConnectorPlacement.EquallySpacedRectSide\",\"uuid\":\"eba5c7b4-5491-40fe-9473-62c3e87abab1\"},{\"content\":{\"connectorIds\":[\"RConn2\",\"RConn3\",\"RConn4\",\"RConn5\"],\"side\":\"BOTTOM\"},\"type\":\"ConnectorPlacement.EquallySpacedRectSide\",\"uuid\":\"126f278d-948c-406c-a2e7-d82f3e8f35fe\"},{\"content\":{\"connectorIds\":[],\"side\":\"HIDDEN\"},\"type\":\"ConnectorPlacement.EquallySpacedRectSide\",\"uuid\":\"f8a4188e-0920-4c7d-8ad7-510b24ee9f78\"}]},\"type\":\"ConnectorPlacement.EquallySpacedConnector\",\"uuid\":\"a41928b5-0f70-4e7a-bf00-47853bb208e5\"}],\"packageUris\":[\"http://schema.mathworks.com/mf0/Connector/R2020b\"],\"version\":\"1.0\"}"
  F9 : PMIOPort  Side=Left
  L4 : PMIOPort  Port=2  Side=Left
  L3 : PMIOPort  Port=3  Side=Left
  L2 : PMIOPort  Port=4  Side=Left
  L1 : PMIOPort  Port=5  Side=Left
  M1 : PMIOPort  Port=6  Side=Right
  M2 : PMIOPort  Port=7  Side=Right
  M3 : PMIOPort  Port=8  Side=Right
  M4 : PMIOPort  Port=9  Side=Right
  connections:
  M2/RConn1 -- whole_batt_base_1_RIGID/LConn3
  Curent_RaspNavBase_1_RIGID/LConn1 -- whole_batt_base_1_RIGID/RConn1
  M3/RConn1 -- whole_batt_base_1_RIGID/LConn4
  M1/RConn1 -- whole_batt_base_1_RIGID/LConn2
  M4/RConn1 -- whole_batt_base_1_RIGID/LConn5
  F9/RConn1 -- whole_batt_base_1_RIGID/LConn1
  L1/RConn1 -- whole_batt_base_1_RIGID/RConn5
  L2/RConn1 -- whole_batt_base_1_RIGID/RConn4
  L3/RConn1 -- whole_batt_base_1_RIGID/RConn3
  L4/RConn1 -- whole_batt_base_1_RIGID/RConn2

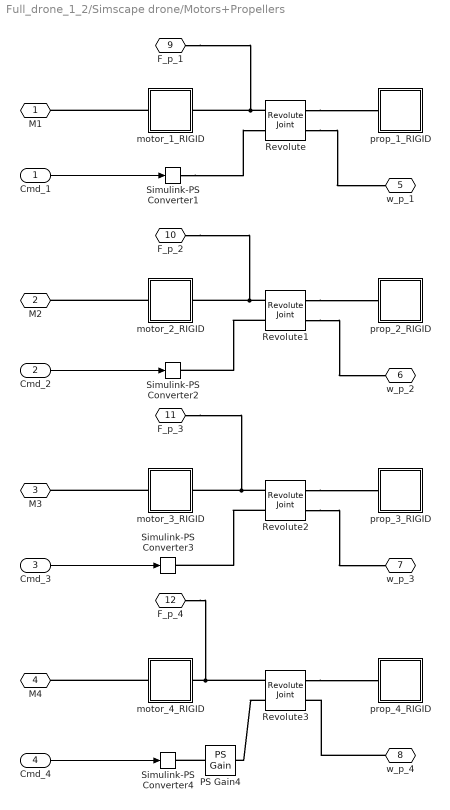
== system Full_drone_1_2/Simscape drone/Motors+Propellers ==
  Cmd_1 : Inport
  Cmd_2 : Inport  Port=2
  Cmd_3 : Inport  Port=3
  Cmd_4 : Inport  Port=4
  PS Gain4 : fl_lib/Physical Signals/Functions/PS Gain  gain=-1
  Revolute{,1..3} (4 alike) : sm_lib/Joints/Revolute Joint  JointMode=Normal  SenseConstraintForce=off  SenseConstraintForceX=off  SenseConstraintForceY=off  SenseConstraintForceZ=off  SenseConstraintTorque=off  SenseConstraintTorqueX=off  SenseConstraintTorqueY=off  SenseConstraintTorqueZ=off  SenseTotalForce=off  SenseTotalForceX=off  SenseTotalForceY=off  SenseTotalForceZ=off  SenseTotalTorque=off  SenseTotalTorqueX=off  SenseTotalTorqueY=off  SenseTotalTorqueZ=off  CompositeWrenchDir=FollowerOnBase  CompositeWrenchFrame=BaseFrame  EquilibriumPosition=0  EquilibriumPositionUnits=deg  SpringStiffness=0  SpringStiffnessUnits=N*m/deg  DampingCoefficient=5e-7  DampingCoefficientUnits=N*m/(deg/s)  TorqueActuationMode=InputTorque  MotionActuationMode=ComputedMotion  SensePosition=off  SenseVelocity=on  SenseAcceleration=off  SenseTorqueForce=off  SenseLowerLimitTorqueForce=off  SenseUpperLimitTorqueForce=off  LowerLimitSpecify=off  LowerLimitBound=-90  LowerLimitBoundUnits=deg  LowerLimitStiffness=1e4  LowerLimitStiffnessUnits=N*m/deg  LowerLimitDamping=10  LowerLimitDampingUnits=N*m/(deg/s)  LowerLimitTransitionRegionWidth=0.1  LowerLimitTransitionRegionWidthUnits=deg  UpperLimitSpecify=off  UpperLimitBound=90  UpperLimitBoundUnits=deg  UpperLimitStiffness=1e4  UpperLimitStiffnessUnits=N*m/deg  UpperLimitDamping=10  UpperLimitDampingUnits=N*m/(deg/s)  UpperLimitTransitionRegionWidth=0.1  UpperLimitTransitionRegionWidthUnits=deg  PositionTargetSpecify=on  PositionTargetPriority=Low  PositionTargetValue=smiData.RevoluteJoint(1).Rz.Pos  PositionTargetValueUnits=deg  VelocityTargetSpecify=off  VelocityTargetPriority=High  VelocityTargetValue=0  VelocityTargetValueUnits=deg/s
  Simulink-PS Converter{1..4} (4 alike) : nesl_utility/Simulink-PS Converter  PhysicalDomain=network_engine_domain  SubClassName=ps_input  LeftPortType=input  RightPortType=output  PseudoPeriodic=off  Frequencies=[]  NoiseDistribution=none  NoiseParameters=[]  Unit=N*m  AffineConversion=off  FilteringAndDerivatives=provide  SimscapeFilterOrder=1  InputFilterTimeConstant=0.001  UdotUserProvided=0
  motor_1_RIGID : Subsystem
  motor_2_RIGID : Subsystem
  motor_3_RIGID : Subsystem
  motor_4_RIGID : Subsystem
  prop_1_RIGID : Subsystem
  prop_2_RIGID : Subsystem
  prop_3_RIGID : Subsystem
  prop_4_RIGID : Subsystem
  M1 : PMIOPort  Side=Left
  M2 : PMIOPort  Port=2  Side=Left
  M3 : PMIOPort  Port=3  Side=Left
  M4 : PMIOPort  Port=4  Side=Left
  w_p_1 : PMIOPort  Port=5  Side=Right
  w_p_2 : PMIOPort  Port=6  Side=Right
  w_p_3 : PMIOPort  Port=7  Side=Right
  w_p_4 : PMIOPort  Port=8  Side=Right
  F_p_1 : PMIOPort  Port=9  Side=Right
  F_p_2 : PMIOPort  Port=10  Side=Right
  F_p_3 : PMIOPort  Port=11  Side=Right
  F_p_4 : PMIOPort  Port=12  Side=Right
  wires:
  Cmd_2/1 -> Simulink-PS Converter2/1
  Cmd_3/1 -> Simulink-PS Converter3/1
  Cmd_4/1 -> Simulink-PS Converter4/1
  Cmd_1/1 -> Simulink-PS Converter1/1
  connections:
  Revolute3/RConn1 -- prop_4_RIGID/LConn1
  Revolute1/RConn2 -- w_p_2/RConn1
  F_p_2/RConn1 -- Revolute1/LConn1 -- motor_2_RIGID/RConn1
  Revolute/LConn1 -- F_p_1/RConn1 -- motor_1_RIGID/RConn1
  Revolute/RConn1 -- prop_1_RIGID/LConn1
  F_p_4/RConn1 -- Revolute3/LConn1 -- motor_4_RIGID/RConn1
  Revolute1/RConn1 -- prop_2_RIGID/LConn1
  F_p_3/RConn1 -- Revolute2/LConn1 -- motor_3_RIGID/LConn1
  Revolute2/RConn1 -- prop_3_RIGID/RConn1
  motor_2_RIGID/LConn1 -- M2/RConn1
  Revolute3/LConn2 -- PS Gain4/RConn1
  motor_1_RIGID/LConn1 -- M1/RConn1
  Revolute2/RConn2 -- w_p_3/RConn1
  Revolute/RConn2 -- w_p_1/RConn1
  motor_4_RIGID/LConn1 -- M4/RConn1
  motor_3_RIGID/RConn1 -- M3/RConn1
  w_p_4/RConn1 -- Revolute3/RConn2
  Simulink-PS Converter1/RConn1 -- Revolute/LConn2
  Revolute1/LConn2 -- Simulink-PS Converter2/RConn1
  Revolute2/LConn2 -- Simulink-PS Converter3/RConn1
  PS Gain4/LConn1 -- Simulink-PS Converter4/RConn1

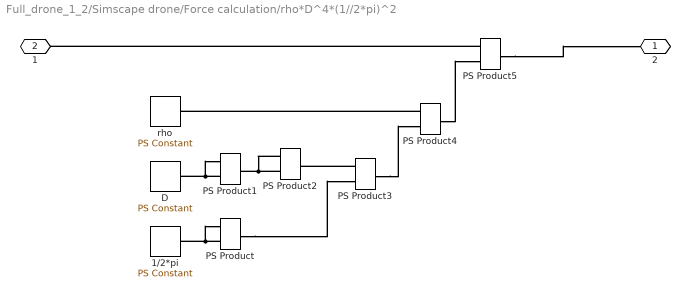
== system Full_drone_1_2/Simscape drone/Force calculation/rho*D^4*(1//2*pi)^2 ==
  1/2*pi : fl_lib/Physical Signals/Sources/PS Constant  constant=1/(2*pi) 1/rad
  D : fl_lib/Physical Signals/Sources/PS Constant  constant=0.12 m
  PS Product{,1..5} (6 alike) : fl_lib/Physical Signals/Functions/PS Product
  rho : fl_lib/Physical Signals/Sources/PS Constant  constant=1.225 kg/m^3
  2 : PMIOPort  Side=Right
  1 : PMIOPort  Port=2  Side=Left
  connections:
  PS Product3/RConn1 -- PS Product4/LConn2
  PS Product/RConn1 -- PS Product3/LConn2
  PS Product5/LConn1 -- 1/RConn1
  PS Product4/RConn1 -- PS Product5/LConn2
  PS Product2/LConn2 -- PS Product2/LConn1 -- PS Product1/RConn1
  PS Product1/LConn2 -- PS Product1/LConn1 -- D/RConn1
  PS Product/LConn2 -- PS Product/LConn1 -- 1/2*pi/RConn1
  PS Product4/LConn1 -- rho/RConn1
  PS Product3/LConn1 -- PS Product2/RConn1
  PS Product5/RConn1 -- 2/RConn1

== system Full_drone_1_2/Simscape drone/Landers/lander_1_RIGID ==
  Brick Solid : sm_lib/Body Elements/Brick Solid  GraphicAmbientColor=[0.15 0.15 0.15 1.0]  BasedOnType=Density  BrickDimensions=[0.022 0.004 0.025]  BrickDimensionUnits=m  CenterOfMass=[0 0 0]  CenterOfMassUnits=m  GraphicDiffuseColor=[0.5 0.5 0.5]  Density=0  DensityUnits=kg/m^3  DoExposeReferenceFrame=off  GraphicEmissiveColor=[0.0 0.0 0.0 1.0]  ExportEntireGeometry=on  SerializedFrames=<Frames><Frame><Id>Frame1</Id><Value><Name>F1</Name><Origin><Source>GeometricFeature</Source><FeatureName>+z surface</FeatureName></Origin><PrimaryAxis><DefinedDirection>+Z</DefinedDirection><Source>ReferenceFrame</Source><SourceDirection>+Z</SourceDirection><FeatureName></FeatureName></PrimaryAxis><SecondaryAxis><DefinedDirection>+X</DefinedDirection><Source>ReferenceFrame</Source><SourceDirection>+X</SourceDirection><FeatureName></FeatureName></SecondaryAxis></Value></Frame></Frames>  MarkerShape=Sphere  MarkerSize=10  GraphicType=FromGeometry  InertiaType=CalculateFromGeometry  Mass=smiData.Solid(3).mass  MassUnits=kg  MomentsOfInertia=[1 1 1]  MomentsOfInertiaUnits=kg*m^2  GraphicOpacity=1.0  ProductsOfInertia=[0 0 0]  ProductsOfInertiaUnits=kg*m^2  GraphicShininess=75  GraphicSpecularColor=[0.5 0.5 0.5 1.0]  GraphicVisPropType=SimpleVisualProperties
  ReferenceFrame : sm_lib/Frames and Transforms/Reference Frame
  Solid : sm_lib/Body Elements/File Solid  ExtGeomFileName=lander_Default_sldprt.STEP  UnitType=FromFile  ExtGeomFileUnits=m  StepReaderType=HEX  ExportConvexHullGeometry=off  InertiaType=Custom  Mass=smiData.Solid(3).mass  MassUnits=kg  CenterOfMass=smiData.Solid(3).CoM  CenterOfMassUnits=mm  MomentsOfInertia=smiData.Solid(3).MoI  MomentsOfInertiaUnits=kg*mm^2  ProductsOfInertia=smiData.Solid(3).PoI  ProductsOfInertiaUnits=kg*mm^2  BasedOnType=DensityFromFile  Density=1000  DensityUnits=kg/m^3  DoExposeReferenceFrame=on  SerializedFrames=<Frames/>  GraphicType=FromGeometry  MarkerShape=Sphere  MarkerSize=10  GraphicVisPropType=SimpleVisualProperties  GraphicDiffuseColor=smiData.Solid(3).color  GraphicSpecularColor=[0.5 0.5 0.5 1.0]  GraphicAmbientColor=[0.15 0.15 0.15 1.0]  GraphicEmissiveColor=[0.0 0.0 0.0 1.0]  GraphicShininess=75  GraphicOpacity=smiData.Solid(3).opacity
  Transform : sm_lib/Frames and Transforms/Rigid Transform  TranslationMethod=Cartesian  TranslationStandardOffset=0  TranslationLengthUnit=mm  TranslationStandardAxis=+Z  TranslationCartesianOffset=smiData.RigidTransform(18).translation  TranslationROffset=0  TranslationROffsetUnits=m  TranslationZOffset=0  TranslationZOffsetUnits=m  TranslationThetaOffset=0  TranslationThetaOffsetUnits=deg  RotationMethod=ArbitraryAxis  RotationAngleUnits=rad  RotationStandardAxis=+Z  RotationAngle=smiData.RigidTransform(18).angle  RotationArbitraryAxis=smiData.RigidTransform(18).axis  FollAlignAxisA=+X  BaseAlignAxisA=+Y  FollAlignAxisB=+Y  BaseAlignAxisB=+Z  RotationSequenceAxes=FollowerAxes  RotationSequence=XYX  RotationSequenceAngles=[0 0 0]  RotationSequenceAnglesUnits=deg  RotationMatrix=[1 0 0; 0 1 0; 0 0 1]
  F : PMIOPort  Side=Left
  F5 : PMIOPort  Port=2  Side=Right
  connections:
  F5/RConn1 -- Brick Solid/RConn1
  ReferenceFrame/RConn1 -- Transform/LConn1 -- Brick Solid/LConn1 -- Solid/RConn1
  F/RConn1 -- Transform/RConn1

== system Full_drone_1_2/Simscape drone/Landers/lander_5_RIGID ==
  Brick Solid : sm_lib/Body Elements/Brick Solid  GraphicAmbientColor=[0.15 0.15 0.15 1.0]  BasedOnType=Density  BrickDimensions=[0.022 0.004 0.025]  BrickDimensionUnits=m  CenterOfMass=[0 0 0]  CenterOfMassUnits=m  GraphicDiffuseColor=[0.5 0.5 0.5]  Density=0  DensityUnits=kg/m^3  DoExposeReferenceFrame=off  GraphicEmissiveColor=[0.0 0.0 0.0 1.0]  ExportEntireGeometry=on  SerializedFrames=<Frames><Frame><Id>Frame1</Id><Value><Name>F1</Name><Origin><Source>GeometricFeature</Source><FeatureName>+z surface</FeatureName></Origin><PrimaryAxis><DefinedDirection>+Z</DefinedDirection><Source>ReferenceFrame</Source><SourceDirection>+Z</SourceDirection><FeatureName></FeatureName></PrimaryAxis><SecondaryAxis><DefinedDirection>+X</DefinedDirection><Source>ReferenceFrame</Source><SourceDirection>+X</SourceDirection><FeatureName></FeatureName></SecondaryAxis></Value></Frame></Frames>  MarkerShape=Sphere  MarkerSize=10  GraphicType=FromGeometry  InertiaType=CalculateFromGeometry  Mass=smiData.Solid(3).mass  MassUnits=kg  MomentsOfInertia=[1 1 1]  MomentsOfInertiaUnits=kg*m^2  GraphicOpacity=1.0  ProductsOfInertia=[0 0 0]  ProductsOfInertiaUnits=kg*m^2  GraphicShininess=75  GraphicSpecularColor=[0.5 0.5 0.5 1.0]  GraphicVisPropType=SimpleVisualProperties
  ReferenceFrame : sm_lib/Frames and Transforms/Reference Frame
  Solid : sm_lib/Body Elements/File Solid  ExtGeomFileName=lander_Default_sldprt.STEP  UnitType=FromFile  ExtGeomFileUnits=m  StepReaderType=HEX  ExportConvexHullGeometry=off  InertiaType=Custom  Mass=smiData.Solid(3).mass  MassUnits=kg  CenterOfMass=smiData.Solid(3).CoM  CenterOfMassUnits=mm  MomentsOfInertia=smiData.Solid(3).MoI  MomentsOfInertiaUnits=kg*mm^2  ProductsOfInertia=smiData.Solid(3).PoI  ProductsOfInertiaUnits=kg*mm^2  BasedOnType=DensityFromFile  Density=1000  DensityUnits=kg/m^3  DoExposeReferenceFrame=on  SerializedFrames=<Frames/>  GraphicType=FromGeometry  MarkerShape=Sphere  MarkerSize=10  GraphicVisPropType=SimpleVisualProperties  GraphicDiffuseColor=smiData.Solid(3).color  GraphicSpecularColor=[0.5 0.5 0.5 1.0]  GraphicAmbientColor=[0.15 0.15 0.15 1.0]  GraphicEmissiveColor=[0.0 0.0 0.0 1.0]  GraphicShininess=75  GraphicOpacity=smiData.Solid(3).opacity
  Transform : sm_lib/Frames and Transforms/Rigid Transform  TranslationMethod=Cartesian  TranslationStandardOffset=0  TranslationLengthUnit=mm  TranslationStandardAxis=+Z  TranslationCartesianOffset=smiData.RigidTransform(20).translation  TranslationROffset=0  TranslationROffsetUnits=m  TranslationZOffset=0  TranslationZOffsetUnits=m  TranslationThetaOffset=0  TranslationThetaOffsetUnits=deg  RotationMethod=ArbitraryAxis  RotationAngleUnits=rad  RotationStandardAxis=+Z  RotationAngle=smiData.RigidTransform(20).angle  RotationArbitraryAxis=smiData.RigidTransform(20).axis  FollAlignAxisA=+X  BaseAlignAxisA=+Y  FollAlignAxisB=+Y  BaseAlignAxisB=+Z  RotationSequenceAxes=FollowerAxes  RotationSequence=XYX  RotationSequenceAngles=[0 0 0]  RotationSequenceAnglesUnits=deg  RotationMatrix=[1 0 0; 0 1 0; 0 0 1]
  F : PMIOPort  Side=Left
  F1 : PMIOPort  Port=2  Side=Right
  connections:
  ReferenceFrame/RConn1 -- Transform/LConn1 -- Solid/RConn1 -- Brick Solid/LConn1
  Transform/RConn1 -- F/RConn1
  F1/RConn1 -- Brick Solid/RConn1

== system Full_drone_1_2/Simscape drone/Landers/lander_6_RIGID ==
  Brick Solid : sm_lib/Body Elements/Brick Solid  GraphicAmbientColor=[0.15 0.15 0.15 1.0]  BasedOnType=Density  BrickDimensions=[0.022 0.004 0.025]  BrickDimensionUnits=m  CenterOfMass=[0 0 0]  CenterOfMassUnits=m  GraphicDiffuseColor=[0.5 0.5 0.5]  Density=0  DensityUnits=kg/m^3  DoExposeReferenceFrame=off  GraphicEmissiveColor=[0.0 0.0 0.0 1.0]  ExportEntireGeometry=on  SerializedFrames=<Frames><Frame><Id>Frame1</Id><Value><Name>F1</Name><Origin><Source>GeometricFeature</Source><FeatureName>+z surface</FeatureName></Origin><PrimaryAxis><DefinedDirection>+Z</DefinedDirection><Source>ReferenceFrame</Source><SourceDirection>+Z</SourceDirection><FeatureName></FeatureName></PrimaryAxis><SecondaryAxis><DefinedDirection>+X</DefinedDirection><Source>ReferenceFrame</Source><SourceDirection>+X</SourceDirection><FeatureName></FeatureName></SecondaryAxis></Value></Frame></Frames>  MarkerShape=Sphere  MarkerSize=10  GraphicType=FromGeometry  InertiaType=CalculateFromGeometry  Mass=smiData.Solid(3).mass  MassUnits=kg  MomentsOfInertia=[1 1 1]  MomentsOfInertiaUnits=kg*m^2  GraphicOpacity=1.0  ProductsOfInertia=[0 0 0]  ProductsOfInertiaUnits=kg*m^2  GraphicShininess=75  GraphicSpecularColor=[0.5 0.5 0.5 1.0]  GraphicVisPropType=SimpleVisualProperties
  ReferenceFrame : sm_lib/Frames and Transforms/Reference Frame
  Solid : sm_lib/Body Elements/File Solid  ExtGeomFileName=lander_Default_sldprt.STEP  UnitType=FromFile  ExtGeomFileUnits=m  StepReaderType=HEX  ExportConvexHullGeometry=off  InertiaType=Custom  Mass=smiData.Solid(3).mass  MassUnits=kg  CenterOfMass=smiData.Solid(3).CoM  CenterOfMassUnits=mm  MomentsOfInertia=smiData.Solid(3).MoI  MomentsOfInertiaUnits=kg*mm^2  ProductsOfInertia=smiData.Solid(3).PoI  ProductsOfInertiaUnits=kg*mm^2  BasedOnType=DensityFromFile  Density=1000  DensityUnits=kg/m^3  DoExposeReferenceFrame=on  SerializedFrames=<Frames/>  GraphicType=FromGeometry  MarkerShape=Sphere  MarkerSize=10  GraphicVisPropType=SimpleVisualProperties  GraphicDiffuseColor=smiData.Solid(3).color  GraphicSpecularColor=[0.5 0.5 0.5 1.0]  GraphicAmbientColor=[0.15 0.15 0.15 1.0]  GraphicEmissiveColor=[0.0 0.0 0.0 1.0]  GraphicShininess=75  GraphicOpacity=smiData.Solid(3).opacity
  Transform : sm_lib/Frames and Transforms/Rigid Transform  TranslationMethod=Cartesian  TranslationStandardOffset=0  TranslationLengthUnit=mm  TranslationStandardAxis=+Z  TranslationCartesianOffset=smiData.RigidTransform(22).translation  TranslationROffset=0  TranslationROffsetUnits=m  TranslationZOffset=0  TranslationZOffsetUnits=m  TranslationThetaOffset=0  TranslationThetaOffsetUnits=deg  RotationMethod=ArbitraryAxis  RotationAngleUnits=rad  RotationStandardAxis=+Z  RotationAngle=smiData.RigidTransform(22).angle  RotationArbitraryAxis=smiData.RigidTransform(22).axis  FollAlignAxisA=+X  BaseAlignAxisA=+Y  FollAlignAxisB=+Y  BaseAlignAxisB=+Z  RotationSequenceAxes=FollowerAxes  RotationSequence=XYX  RotationSequenceAngles=[0 0 0]  RotationSequenceAnglesUnits=deg  RotationMatrix=[1 0 0; 0 1 0; 0 0 1]
  F : PMIOPort  Side=Left
  F1 : PMIOPort  Port=2  Side=Right
  connections:
  ReferenceFrame/RConn1 -- Brick Solid/LConn1 -- Solid/RConn1 -- Transform/LConn1
  Transform/RConn1 -- F/RConn1
  F1/RConn1 -- Brick Solid/RConn1
